simulink model "IdentPlanar"  (Simulink 7.9)
settings: Solver=FixedStepDiscrete  StartTime=0.0  StopTime=3600  FixedStep=1/Fs  RelTol=1e-3
values from neighbouring files (symbols this model uses):
  abs2deg_s1 = (s1max-s1min)/(s1maxabs-s1minabs)    (= 0.280034572169)    [Alex_init_const_wrist.m]
  abs2deg_s2 = (s2max-s2min)/(s2maxabs-s2minabs)    (= 0.060826446281)    [Alex_init_const_wrist.m]
  c1x = 0    [Alex_init_const_shoulderelbow.m]
  c1y = 0    [Alex_init_const_shoulderelbow.m]
  c1z = 0    [Alex_init_const_shoulderelbow.m]
  c2x = 1.79e-3    (= 0.00179)    [Alex_init_const_shoulderelbow.m]
  c2y = 0    [Alex_init_const_shoulderelbow.m]
  c2z = 228.5e-3    (= 0.2285)    [Alex_init_const_shoulderelbow.m]
  c3x = 0    [Alex_init_const_shoulderelbow.m]
  c3y = 0    [Alex_init_const_shoulderelbow.m]
  c3z = 0    [Alex_init_const_shoulderelbow.m]
  c4x = 1.91e-3    (= 0.00191)    [Alex_init_const_shoulderelbow.m]
  c4y = 0    [Alex_init_const_shoulderelbow.m]
  c4z = 163e-3    (= 0.163)    [Alex_init_const_shoulderelbow.m]
  c5x = 0    [Alex_init_const_shoulderelbow.m]
  c5y = 0    [Alex_init_const_shoulderelbow.m]
  c5z = 0    [Alex_init_const_shoulderelbow.m]
  deg_rad = pi/180    (= 0.0174532925199)    [Alex_init_const_shoulderelbow.m]
  E1initial = qtot(initialtime*Fs,1)    [Alex_init_const_shoulderelbow.m]
  Fs = 1000    [Alex_init_const_wrist.m]
  initialtime = 5    [Alex_init_const_shoulderelbow.m]
  Ll = 324.6e-3    (= 0.3246)    [Alex_init_const_shoulderelbow.m]
  Lu = 332.3e-3    (= 0.3323)    [Alex_init_const_shoulderelbow.m]
  ml = 1.649    [Alex_init_const_shoulderelbow.m]
  mu = 2.804    [Alex_init_const_shoulderelbow.m]
  Nm2mA_e1 = 1000/(Kv_e1*GRe1)    [Alex_init_const_shoulderelbow.m]
  Nm2mA_s1 = 1000/(Kv_s1*GR_s1)    [Alex_init_const_shoulderelbow.m]
  Nm2mA_s2 = 1000/(Kv_s2*GR_s2)    [Alex_init_const_shoulderelbow.m]
  Nm2mA_s3 = 1000/(Kv_s3*GR_s3)    [Alex_init_const_shoulderelbow.m]
  S2initial = qtot(initialtime*Fs,2)    [Alex_init_const_shoulderelbow.m]
  s2maxabs = 3420    [Alex_init_const_wrist.m]
  s2minabs = 395    [Alex_init_const_wrist.m]
  Ts = 1/Fs    [Alex_init_const_shoulderelbow.m]    (also in Alex_init_const_wrist.m = 0.001)
undefined symbols (not defined in the file or in its folder): abs2deg_e1, abs2deg_e2, abs2deg_s3, CPT_s1, CPT_s2, CPTe1, CPTe2, CPTs3, e2maxabs, e2minabs, GR_s1, GR_s2, GR_s3, GRe1, GRe2, ilim_e1, ilim_e2, ilim_s1, ilim_s2, ilim_s3, Kd_e1, Kd_e2, Kd_s1, Kd_s2, Kd_s3, Ki_e1, Ki_e2, Ki_s1, Ki_s2, Ki_s3, s1zeroabs, s3maxabs, s3minabs
libraries: SERGIOarm x10, simulink x4, SERGIO_Lib x2
settings Model: Creator=root  LastModifiedBy=root  SimulationMode=external  ExtModeTrigElement=1  ExtModeTrigDuration=3910  ExtModeAutoUpdateStatusClock=off
settings DataIOCC: LimitDataPoints=off  MaxDataPoints=4000*3600  SaveOutput=off  SignalLogging=off  SaveTime=off
settings OptimizationCC: BlockReduction=off  BooleanDataType=off  InitFltsAndDblsToZero=on
settings DebuggingCC: SaveWithParameterizedLinksMsg=none  SignalResolutionControl=TryResolveAllWithWarning  SolverPrmCheckMsg=none  MultiTaskDSMMsg=warning  MultiTaskCondExecSysMsg=none  FcnCallInpInsideContextMsg=Use local settings  StrictBusMsg=None
settings HardwareCC: TargetBitPerLong=64  TargetBitPerPointer=64  TargetEndianess=LittleEndian  TargetWordSize=64  TargetHWDeviceType=MATLAB Host
settings ModelReferenceCC: ModelReferencePassRootInputsByReference=off
settings RTWCC: SystemTargetFile=mttarget.tlc  MakeCommand="make_rtw CC=\"ccache gcc\" OPTS=\"-DNETIF_ID=0 -D_GNU_SOURCE -DPRIO=99\""  TemplateMakefile=mt_unix.tmf  Description=Robocup Real-Time Motion Target  ProcessScript=mttarget_make_rtw_hook  IncludeERTFirstTime=on  RTWCompilerOptimization=Custom  RTWCustomCompilerOptimizations=-O2 -g -W
settings RTWCC: CustomInclude=|
  | /usr/local/include/soem
  | /usr/local/include/timer_posix
settings RTWCC: CustomLibrary=|
  | /usr/local/lib/libsoem.so
  | /usr/lib/libtimer_posix.so
settings GRTTargetCC: LogVarNameModifier=none  ExtMode=on

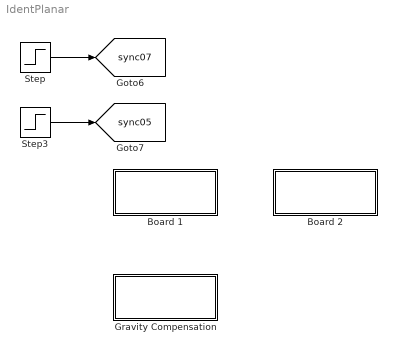
== system IdentPlanar ==
  Board 1 : Subsystem
  Board 2 : Subsystem
  Gravity Compensation : Subsystem
  Step : Step  Time=0.7  Before=1  After=0  SampleTime=0
  Step3 : Step  Time=0.5  Before=1  After=0  SampleTime=0
  tag scope: sync05=global, sync07=global
  wires:
  Step/1 -> [sync07]
  Step3/1 -> [sync05]

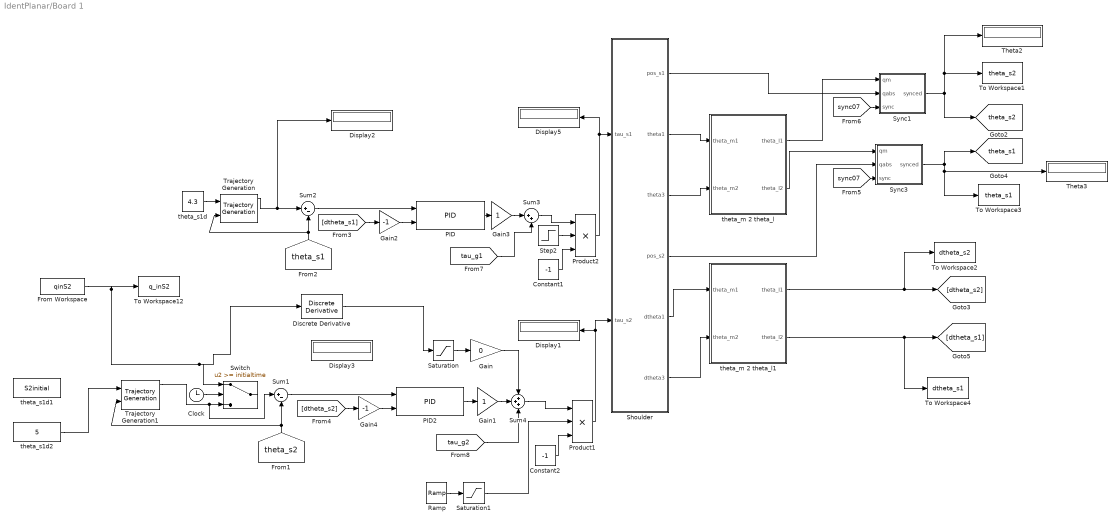
== system IdentPlanar/Board 1 ==
  Clock : Clock
  Constant1 : Constant  Value=-1
  Constant2 : Constant  Value=-1
  Discrete Derivative : simulink/Discrete/Discrete Derivative  gainval=1.0  ICPrevScaledInput=0.0  InputProcessing=Inherited  OutMin=[]  OutMax=[]  OutDataType=fixdt(1, 16)  OutScaling=2^-10  DoSatur=off
  Display{1..3,5} (4 alike) : Display
  From Workspace : FromWorkspace  VariableName=qinS2  SampleTime=1/Fs  OutputAfterFinalValue=Holding final value
  Gain : Gain  Gain=0
  Gain1 : Gain
  Gain2 : Gain  Gain=-1
  Gain3 : Gain
  Gain4 : Gain  Gain=-1
  PID : SERGIOarm/PID  Kc=Kc_s1  Ki=Ki_s1  Kd=Kd_s1  uplim=ilim_s1  lowlim=-ilim_s1  Ts=Ts
  PID2 : SERGIOarm/PID  Kc=Kc_s2  Ki=Ki_s2  Kd=Kd_s2  uplim=ilim_s2  lowlim=-ilim_s2  Ts=Ts
  Product1 : Product  Inputs=3  RndMeth=Zero
  Product2 : Product  Inputs=3  RndMeth=Zero
  Ramp : simulink/Sources/Ramp  slope=1  start=0.8  X0=0
  Saturation : Saturate  UpperLimit=1  LowerLimit=-1
  Saturation1 : Saturate  UpperLimit=1  LowerLimit=0
  Shoulder : Subsystem
  Step2 : Step  Time=0.8  SampleTime=0
  Sum1 : Sum  Inputs=|+-
  Sum2 : Sum  Inputs=|+-
  Sum3 : Sum  Inputs=|++
  Sum4 : Sum  Inputs=+++
  Switch : Switch  Threshold=initialtime
  Sync1 : Subsystem
  Sync3 : Subsystem
  Theta2 : Display
  Theta3 : Display
  To Workspace1 : ToWorkspace  VariableName=theta_s2  SampleTime=-1
  To Workspace12 : ToWorkspace  VariableName=q_inS2  SampleTime=-1
  To Workspace2 : ToWorkspace  VariableName=dtheta_s2  SampleTime=-1
  To Workspace3 : ToWorkspace  VariableName=theta_s1  SampleTime=-1
  To Workspace4 : ToWorkspace  VariableName=dtheta_s1  SampleTime=-1
  Trajectory Generation : SERGIOarm/Trajectory Generation  Vmax=Vmax  Amax=Amax  dif_in=0.1
  Trajectory Generation1 : SERGIOarm/Trajectory Generation  Vmax=Vmax  Amax=Amax  dif_in=1
  theta_m 2 theta_l : Subsystem
  theta_m 2 theta_l1 : Subsystem
  theta_s1d : Constant  Value=4.3
  theta_s1d1 : Constant  Value=S2initial
  theta_s1d2 : Constant  Value=5
  tag scope: theta_s1=global, theta_s2=global
  wires:
  Product2/1 -> Display5/1, Shoulder/1(tau_s1)
  theta_m 2 theta_l/1(theta_l1) -> Sync1/1(qm)
  theta_m 2 theta_l/2(theta_l2) -> Sync3/1(qm)
  Shoulder/6(dtheta3) -> theta_m 2 theta_l1/2(theta_m2)
  theta_m 2 theta_l1/1(theta_l1) -> [dtheta_s2], To Workspace2/1
  theta_m 2 theta_l1/2(theta_l2) -> [dtheta_s1], To Workspace4/1
  Step2/1 -> Product2/2
  Constant1/1 -> Product2/3
  [dtheta_s1] -> Gain2/1
  Product1/1 -> Display1/1, Shoulder/2(tau_s2)
  Saturation1/1 -> Product1/2
  Constant2/1 -> Product1/3
  [dtheta_s2] -> Gain4/1
  Shoulder/5(dtheta1) -> theta_m 2 theta_l1/1(theta_m1)
  Shoulder/2(theta1) -> theta_m 2 theta_l/1(theta_m1)
  Shoulder/3(theta3) -> theta_m 2 theta_l/2(theta_m2)
  Shoulder/4(pos_s2) -> Sync3/2(qabs)
  Sync3/1(synced) -> [theta_s1], Theta3/1, To Workspace3/1
  [sync07] -> Sync3/3(sync)
  Shoulder/1(pos_s1) -> Sync1/2(qabs)
  [sync07] -> Sync1/3(sync)
  Sync1/1(synced) -> [theta_s2], To Workspace1/1, Theta2/1
  Gain3/1 -> Sum3/1
  [tau_g1] -> Sum3/2
  PID/1 -> Gain3/1
  Sum3/1 -> Product2/1
  PID2/1 -> Gain1/1
  Sum4/1 -> Product1/1
  Trajectory Generation/1 -> Sum2/1, Display2/1
  Sum2/1 -> PID/1
  [theta_s1] -> Sum2/2, Trajectory Generation/2
  theta_s1d/1 -> Trajectory Generation/1
  Sum1/1 -> PID2/1
  [theta_s2] -> Sum1/2, Trajectory Generation1/2
  Gain2/1 -> PID/2
  Gain4/1 -> PID2/2
  From Workspace/1 -> To Workspace12/1, Discrete Derivative/1, Switch/1
  Discrete Derivative/1 -> Saturation/1
  Saturation/1 -> Gain/1
  Gain/1 -> Sum4/1
  Gain1/1 -> Sum4/2
  [tau_g2] -> Sum4/3
  Trajectory Generation1/1 -> Switch/3, Sum1/1
  Clock/1 -> Switch/2
  Ramp/1 -> Saturation1/1
  theta_s1d2/1 -> Trajectory Generation1/1

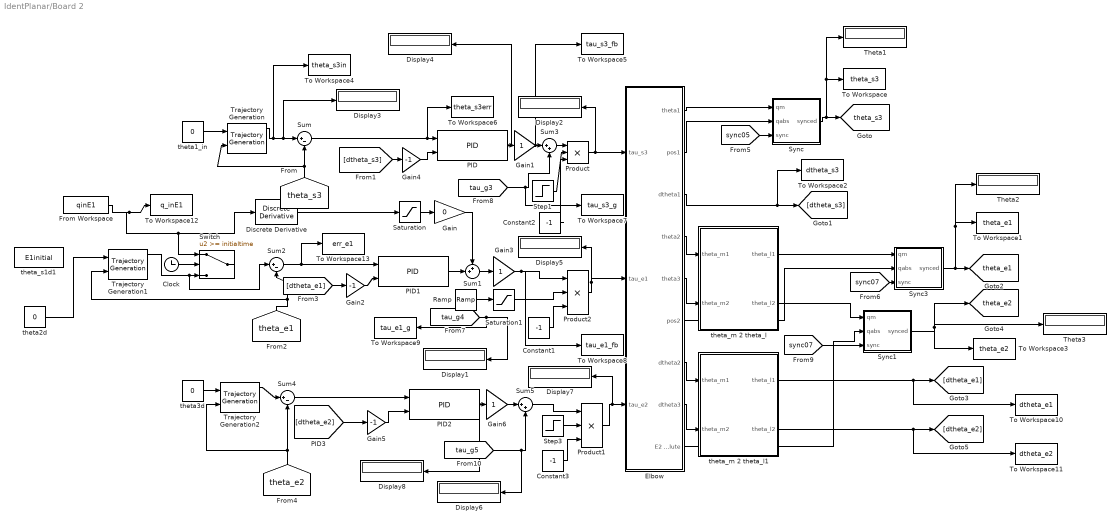
== system IdentPlanar/Board 2 ==
  Clock : Clock
  Constant1 : Constant  Value=-1
  Constant2 : Constant  Value=-1
  Constant3 : Constant  Value=-1
  Discrete Derivative : simulink/Discrete/Discrete Derivative  gainval=1.0  ICPrevScaledInput=0.0  InputProcessing=Inherited  OutMin=[]  OutMax=[]  OutDataType=fixdt(1, 16)  OutScaling=2^-10  DoSatur=off
  Display{1..8} (8 alike) : Display
  Elbow : Subsystem
  From Workspace : FromWorkspace  VariableName=qinE1  SampleTime=1/Fs  OutputAfterFinalValue=Holding final value
  Gain : Gain  Gain=0
  Gain1 : Gain
  Gain2 : Gain  Gain=-1
  Gain3 : Gain
  Gain4 : Gain  Gain=-1
  Gain5 : Gain  Gain=-1
  Gain6 : Gain
  PID : SERGIOarm/PID  Kc=Kc_s3  Ki=Ki_s3  Kd=Kd_s3  uplim=ilim_s3  lowlim=-ilim_s3  Ts=Ts
  PID1 : SERGIOarm/PID  Kc=Kc_e1  Ki=Ki_e1  Kd=Kd_e1  uplim=ilim_e1  lowlim=-ilim_e1  Ts=Ts
  PID2 : SERGIOarm/PID  Kc=Kc_e2  Ki=Ki_e2  Kd=Kd_e2  uplim=ilim_e2  lowlim=-ilim_e2  Ts=Ts
  Product : Product  Inputs=3  RndMeth=Zero
  Product1 : Product  Inputs=3  RndMeth=Zero
  Product2 : Product  Inputs=3  RndMeth=Zero
  Ramp : simulink/Sources/Ramp  slope=1  start=0.8  X0=0
  Saturation : Saturate  UpperLimit=1  LowerLimit=-1
  Saturation1 : Saturate  UpperLimit=1  LowerLimit=0
  Step1 : Step  Time=0.8  SampleTime=0
  Step3 : Step  Time=0.8  SampleTime=0
  Sum : Sum  Inputs=|+-
  Sum1 : Sum  Inputs=++|
  Sum2 : Sum  Inputs=|+-
  Sum3 : Sum  Inputs=|++
  Sum4 : Sum  Inputs=|+-
  Sum5 : Sum  Inputs=|++
  Switch : Switch  Threshold=initialtime
  Sync : Subsystem
  Sync1 : Subsystem
  Sync3 : Subsystem
  Theta1 : Display
  Theta2 : Display
  Theta3 : Display
  To Workspace : ToWorkspace  VariableName=theta_s3  SampleTime=-1
  To Workspace1 : ToWorkspace  VariableName=theta_e1  SampleTime=-1
  To Workspace10 : ToWorkspace  VariableName=dtheta_e1  SampleTime=-1
  To Workspace11 : ToWorkspace  VariableName=dtheta_e2  SampleTime=-1
  To Workspace12 : ToWorkspace  VariableName=q_inE1  SampleTime=-1
  To Workspace13 : ToWorkspace  VariableName=err_e1  SampleTime=-1
  To Workspace2 : ToWorkspace  VariableName=dtheta_s3  SampleTime=-1
  To Workspace3 : ToWorkspace  VariableName=theta_e2  SampleTime=-1
  To Workspace4 : ToWorkspace  VariableName=theta_s3in  SampleTime=-1
  To Workspace5 : ToWorkspace  VariableName=tau_s3_fb  SampleTime=-1
  To Workspace6 : ToWorkspace  VariableName=theta_s3err  SampleTime=-1
  To Workspace7 : ToWorkspace  VariableName=tau_s3_g  SampleTime=-1
  To Workspace8 : ToWorkspace  VariableName=tau_e1_fb  SampleTime=-1
  To Workspace9 : ToWorkspace  VariableName=tau_e1_g  SampleTime=-1
  Trajectory Generation : SERGIOarm/Trajectory Generation  Vmax=Vmax  Amax=Amax  dif_in=1
  Trajectory Generation1 : SERGIOarm/Trajectory Generation  Vmax=Vmax  Amax=Amax  dif_in=0.1
  Trajectory Generation2 : SERGIOarm/Trajectory Generation  Vmax=Vmax  Amax=Amax  dif_in=1
  theta1_in : Constant  Value=0
  theta2d : Constant  Value=0
  theta3d : Constant  Value=0
  theta_m 2 theta_l : Subsystem
  theta_m 2 theta_l1 : Subsystem
  theta_s1d1 : Constant  Value=E1initial
  tag scope: theta_e1=global, theta_e2=global, theta_s3=global
  wires:
  [theta_s3] -> Sum/2, Trajectory Generation/2
  [theta_e1] -> Sum2/2, Trajectory Generation1/2
  Sum4/1 -> PID2/1
  [theta_e2] -> Sum4/2, Trajectory Generation2/2
  Elbow/1(theta1) -> Sync/1(qm)
  Step1/1 -> Product/2
  [sync05] -> Sync/3(sync)
  Sum/1 -> To Workspace6/1, PID/1
  Product2/1 -> Elbow/2(tau_e1), Display5/1
  [dtheta_s3] -> Gain4/1
  Product/1 -> Elbow/1(tau_s3), Display2/1
  Sync/1(synced) -> [theta_s3], To Workspace/1, Theta1/1
  Elbow/2(pos1) -> Sync/2(qabs)
  Elbow/3(dtheta1) -> [dtheta_s3], To Workspace2/1
  Elbow/4(theta2) -> theta_m 2 theta_l/1(theta_m1)
  Elbow/5(theta3) -> theta_m 2 theta_l/2(theta_m2)
  theta_m 2 theta_l/1(theta_l1) -> Sync3/1(qm)
  Elbow/6(pos2) -> Sync3/2(qabs)
  Sync3/1(synced) -> [theta_e1], To Workspace1/1, Theta2/1
  [sync07] -> Sync3/3(sync)
  Elbow/7(dtheta2) -> theta_m 2 theta_l1/1(theta_m1)
  Elbow/8(dtheta3) -> theta_m 2 theta_l1/2(theta_m2)
  theta_m 2 theta_l1/1(theta_l1) -> [dtheta_e1], To Workspace10/1
  theta_m 2 theta_l1/2(theta_l2) -> [dtheta_e2], To Workspace11/1
  Saturation1/1 -> Product2/2
  Constant1/1 -> Product2/3
  [dtheta_e1] -> Gain2/1
  Gain3/1 -> To Workspace8/1, Product2/1
  PID/1 -> Gain1/1, Display4/1
  Gain1/1 -> Sum3/1, To Workspace5/1
  Sum3/1 -> Product/1
  [tau_g3] -> Sum3/2, To Workspace7/1
  Sum2/1 -> PID1/1, To Workspace13/1
  Constant2/1 -> Product/3
  theta1_in/1 -> Trajectory Generation/1
  Gain2/1 -> PID1/2
  Gain4/1 -> PID/2
  theta_m 2 theta_l/2(theta_l2) -> Sync1/1(qm)
  Elbow/9(E2 absolute) -> Sync1/2(qabs)
  [sync07] -> Sync1/3(sync)
  Sync1/1(synced) -> [theta_e2], To Workspace3/1, Theta3/1
  Trajectory Generation2/1 -> Sum4/1
  theta3d/1 -> Trajectory Generation2/1
  Gain5/1 -> PID2/2
  [dtheta_e2] -> Gain5/1
  Step3/1 -> Product1/2
  Constant3/1 -> Product1/3
  Sum5/1 -> Product1/1
  Gain6/1 -> Sum5/1
  [tau_g5] -> Sum5/2, Display6/1
  PID2/1 -> Gain6/1, Display8/1
  Product1/1 -> Elbow/3(tau_e2), Display7/1
  Trajectory Generation/1 -> To Workspace4/1, Sum/1, Display3/1
  From Workspace/1 -> To Workspace12/1, Discrete Derivative/1, Switch/1
  [tau_g4] -> To Workspace9/1, Display1/1
  Saturation/1 -> Gain/1
  Sum1/1 -> Gain3/1
  PID1/1 -> Sum1/2
  Discrete Derivative/1 -> Saturation/1
  Gain/1 -> Sum1/1
  Trajectory Generation1/1 -> Switch/3, Sum2/1
  Clock/1 -> Switch/2
  Ramp/1 -> Saturation1/1
  theta2d/1 -> Trajectory Generation1/1

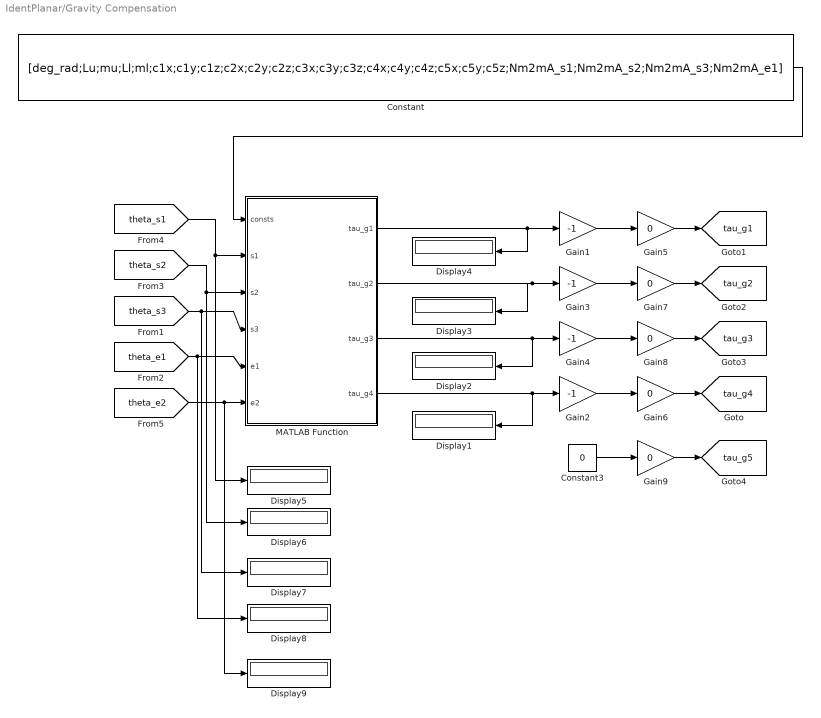
== system IdentPlanar/Gravity Compensation ==
  Constant : Constant  Value=[deg_rad;Lu;mu;Ll;ml;c1x;c1y;c1z;c2x;c2y;c2z;c3x;c3y;c3z;c4x;c4y;c4z;c5x;c5y;c5z;Nm2mA_s1;Nm2mA_s2;Nm2mA_s3;Nm2mA_e1]
  Constant3 : Constant  Value=0
  Display{1..9} (9 alike) : Display
  Gain{1..4} (4 alike) : Gain  Gain=-1
  Gain{5..9} (5 alike) : Gain  Gain=0
  MATLAB Function : MATLAB Function  TreatAsAtomicUnit=on
  tag scope: tau_g1=global, tau_g2=global, tau_g3=global, tau_g4=global, tau_g5=global
  wires:
  [theta_s1] -> Display5/1, MATLAB Function/2(s1)
  [theta_s2] -> Display6/1, MATLAB Function/3(s2)
  [theta_s3] -> MATLAB Function/4(s3), Display7/1
  [theta_e1] -> MATLAB Function/5(e1), Display8/1
  [theta_e2] -> MATLAB Function/6(e2), Display9/1
  Constant/1 -> MATLAB Function/1(consts)
  MATLAB Function/1(tau_g1) -> Display4/1, Gain1/1
  MATLAB Function/2(tau_g2) -> Display3/1, Gain3/1
  MATLAB Function/3(tau_g3) -> Display2/1, Gain4/1
  MATLAB Function/4(tau_g4) -> Display1/1, Gain2/1
  Gain1/1 -> Gain5/1
  Gain3/1 -> Gain7/1
  Gain4/1 -> Gain8/1
  Gain2/1 -> Gain6/1
  Gain5/1 -> [tau_g1]
  Gain7/1 -> [tau_g2]
  Gain8/1 -> [tau_g3]
  Gain6/1 -> [tau_g4]
  Gain9/1 -> [tau_g5]
  Constant3/1 -> Gain9/1

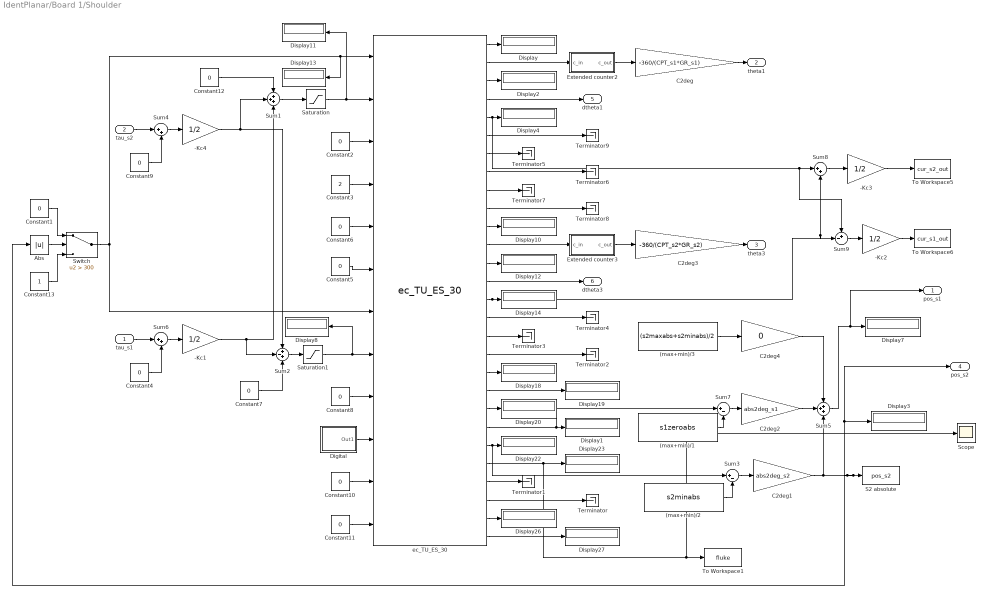
== system IdentPlanar/Board 1/Shoulder ==
  tau_s1 : Inport
  tau_s2 : Inport  Port=2
  (max+min)/1 : Constant  Value=s1zeroabs
  (max+min)/2 : Constant  Value=s2minabs
  (max+min)/3 : Constant  Value=(s2maxabs+s2minabs)/2
  -Kc{1..4} (4 alike) : Gain  Gain=1/2
  Abs : Abs
  C2deg : Gain  Gain=-360/(CPT_s1*GR_s1)
  C2deg1 : Gain  Gain=abs2deg_s2
  C2deg2 : Gain  Gain=abs2deg_s1
  C2deg3 : Gain  Gain=-360/(CPT_s2*GR_s2)
  C2deg4 : Gain  Gain=0
  Constant{1..2,4..12} (11 alike) : Constant  Value=0
  Constant13 : Constant
  Constant3 : Constant  Value=2
  Digital : Subsystem
  Display{,1..4,7..8,10..14,18..20,22..23,26..27} (19 alike) : Display
  Extended counter2 : Subsystem
  Extended counter3 : Subsystem
  S2 absolute : ToWorkspace  VariableName=pos_s2  SampleTime=-1
  Saturation : Saturate  UpperLimit=2400  LowerLimit=-2400
  Saturation1 : Saturate  UpperLimit=2400  LowerLimit=-2400
  Scope : Scope
      settings: TimeRange=10  YMin=0  YMax=350  SampleInput=on
  Sum1 : Sum  Inputs=+++
  Sum2 : Sum  Inputs=+-+
  Sum3 : Sum  Inputs=|+-
  Sum4 : Sum  Inputs=|++
  Sum5 : Sum  Inputs=+++
  Sum6 : Sum  Inputs=|++
  Sum7 : Sum  Inputs=|+-
  Sum8 : Sum  Inputs=|++
  Sum9 : Sum  Inputs=+-|
  Switch : Switch  Criteria=u2 > Threshold  Threshold=300
  Terminator{,1..9} (10 alike) : Terminator
  To Workspace1 : ToWorkspace  VariableName=fluke  SampleTime=-1
  To Workspace5 : ToWorkspace  VariableName=cur_s2_out  SampleTime=-1
  To Workspace6 : ToWorkspace  VariableName=cur_s1_out  SampleTime=-1
  ec_TU_ES_30 : SERGIO_Lib/EtherCAT Blocks/ec_TU_ES_30  link_id=1  slave_num=2  resistance=[0.611+0.45*2, 1.0, 0.611+0.45*2]  kv=[0.0259, 0, 0.0259]  pgain=[4.00, 0.00, 4.00]  igain=[50.00, 0.00, 50.00]  ilimit=[1.0, 1.0, 1.0]  encdir=[1, 1, 1]  encres=[2000, 2000, 2000]  czero=[17230, 8633, 8526]
  pos_s1 : Outport
  theta1 : Outport  Port=2
  theta3 : Outport  Port=3
  pos_s2 : Outport  Port=4
  dtheta1 : Outport  Port=5
  dtheta3 : Outport  Port=6
  wires:
  Constant2/1 -> ec_TU_ES_30/3
  Constant5/1 -> ec_TU_ES_30/6
  Constant8/1 -> ec_TU_ES_30/9
  Digital/1(Out1) -> ec_TU_ES_30/10
  Constant10/1 -> ec_TU_ES_30/11
  Constant11/1 -> ec_TU_ES_30/12
  ec_TU_ES_30/1 -> Display/1
  ec_TU_ES_30/3 -> Display2/1
  ec_TU_ES_30/4 -> dtheta1/1
  ec_TU_ES_30/5 -> Display4/1, Sum8/1, Sum9/1
  ec_TU_ES_30/6 -> Terminator9/1
  ec_TU_ES_30/8 -> Terminator6/1
  ec_TU_ES_30/9 -> Terminator7/1
  ec_TU_ES_30/10 -> Terminator8/1
  ec_TU_ES_30/11 -> Display10/1
  ec_TU_ES_30/13 -> Display12/1
  ec_TU_ES_30/14 -> dtheta3/1
  ec_TU_ES_30/15 -> Display14/1, Sum8/2, Sum9/2
  ec_TU_ES_30/16 -> Terminator4/1
  ec_TU_ES_30/17 -> Terminator3/1
  ec_TU_ES_30/18 -> Terminator2/1
  ec_TU_ES_30/19 -> Display18/1
  ec_TU_ES_30/20 -> Display19/1
  ec_TU_ES_30/21 -> Display20/1
  ec_TU_ES_30/24 -> Display23/1, To Workspace1/1, Scope/1
  ec_TU_ES_30/25 -> Terminator1/1
  ec_TU_ES_30/26 -> Terminator/1
  ec_TU_ES_30/27 -> Display26/1
  ec_TU_ES_30/28 -> Display27/1
  C2deg/1 -> theta1/1
  ec_TU_ES_30/2 -> Extended counter2/1(c_in)
  Extended counter2/1(c_out) -> C2deg/1
  Sum1/1 -> Saturation/1
  Saturation/1 -> ec_TU_ES_30/2, Display11/1
  Sum2/1 -> Saturation1/1
  Saturation1/1 -> ec_TU_ES_30/8, Display8/1
  ec_TU_ES_30/7 -> Terminator5/1
  ec_TU_ES_30/12 -> Extended counter3/1(c_in)
  Extended counter3/1(c_out) -> C2deg3/1
  C2deg3/1 -> theta3/1
  Sum4/1 -> -Kc4/1
  tau_s2/1 -> Sum4/1
  Sum6/1 -> -Kc1/1
  tau_s1/1 -> Sum6/1
  Constant4/1 -> Sum6/2
  ec_TU_ES_30/22 -> Display1/1, Sum7/1
  Constant3/1 -> ec_TU_ES_30/4
  Constant6/1 -> ec_TU_ES_30/5
  Constant12/1 -> Sum1/1
  -Kc4/1 -> Sum1/2, Sum2/1
  -Kc1/1 -> Sum1/3, Sum2/2
  Constant9/1 -> Sum4/2
  Constant7/1 -> Sum2/3
  (max+min)/2/1 -> Sum3/2
  Sum3/1 -> C2deg1/1
  C2deg1/1 -> S2 absolute/1, Abs/1, Display3/1, pos_s2/1, Sum5/3
  ec_TU_ES_30/23 -> Display22/1, Sum3/1
  Switch/1 -> ec_TU_ES_30/7, ec_TU_ES_30/1, Display13/1
  Constant1/1 -> Switch/1
  Abs/1 -> Switch/2
  Constant13/1 -> Switch/3
  Sum5/1 -> Display7/1, pos_s1/1
  (max+min)/3/1 -> C2deg4/1
  C2deg4/1 -> Sum5/1
  C2deg2/1 -> Sum5/2
  (max+min)/1/1 -> Sum7/2
  Sum7/1 -> C2deg2/1
  Sum8/1 -> -Kc3/1
  -Kc3/1 -> To Workspace5/1
  Sum9/1 -> -Kc2/1
  -Kc2/1 -> To Workspace6/1

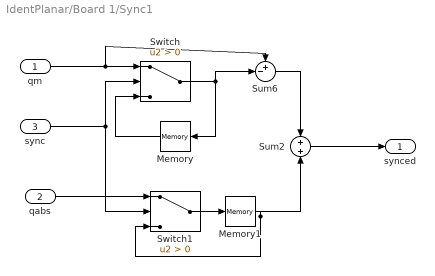
== system IdentPlanar/Board 1/Sync1 ==
  qm : Inport
  qabs : Inport  Port=2
  sync : Inport  Port=3
  Memory : Memory
  Memory1 : Memory
  Sum2 : Sum
  Sum6 : Sum  Inputs=+-|
  Switch : Switch  Criteria=u2 > Threshold
  Switch1 : Switch  Criteria=u2 > Threshold
  synced : Outport
  wires:
  Switch/1 -> Sum6/2, Memory/1
  Memory/1 -> Switch/3
  qm/1 -> Switch/1, Sum6/1
  Sum6/1 -> Sum2/1
  Sum2/1 -> synced/1
  sync/1 -> Switch/2, Switch1/2
  Memory1/1 -> Switch1/3, Sum2/2
  Switch1/1 -> Memory1/1
  qabs/1 -> Switch1/1

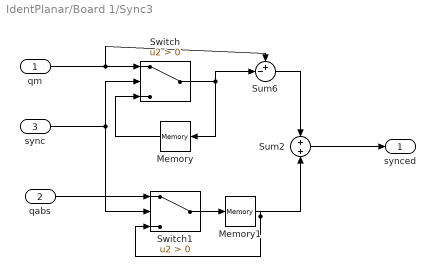
== system IdentPlanar/Board 1/Sync3 ==
  qm : Inport
  qabs : Inport  Port=2
  sync : Inport  Port=3
  Memory : Memory
  Memory1 : Memory
  Sum2 : Sum
  Sum6 : Sum  Inputs=+-|
  Switch : Switch  Criteria=u2 > Threshold
  Switch1 : Switch  Criteria=u2 > Threshold
  synced : Outport
  wires:
  Switch/1 -> Sum6/2, Memory/1
  Memory/1 -> Switch/3
  qm/1 -> Switch/1, Sum6/1
  Sum6/1 -> Sum2/1
  Sum2/1 -> synced/1
  sync/1 -> Switch/2, Switch1/2
  Memory1/1 -> Switch1/3, Sum2/2
  Switch1/1 -> Memory1/1
  qabs/1 -> Switch1/1

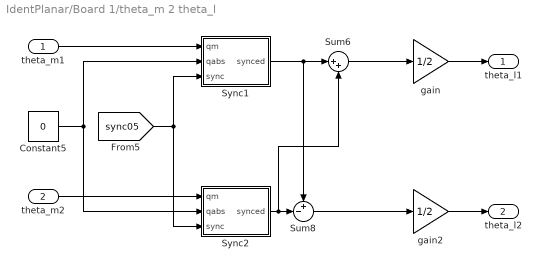
== system IdentPlanar/Board 1/theta_m 2 theta_l ==
  theta_m1 : Inport
  theta_m2 : Inport  Port=2
  Constant5 : Constant  Value=0
  Sum6 : Sum  Inputs=|++
  Sum8 : Sum  Inputs=+-|
  Sync1 : Subsystem
  Sync2 : Subsystem
  gain : Gain  Gain=1/2
  gain2 : Gain  Gain=1/2
  theta_l1 : Outport
  theta_l2 : Outport  Port=2
  wires:
  theta_m2/1 -> Sync2/1(qm)
  theta_m1/1 -> Sync1/1(qm)
  Constant5/1 -> Sync1/2(qabs), Sync2/2(qabs)
  Sync2/1(synced) -> Sum8/2, Sum6/2
  Sync1/1(synced) -> Sum6/1, Sum8/1
  Sum6/1 -> gain/1
  gain/1 -> theta_l1/1
  gain2/1 -> theta_l2/1
  [sync05] -> Sync1/3(sync), Sync2/3(sync)
  Sum8/1 -> gain2/1

== system IdentPlanar/Board 1/theta_m 2 theta_l1 ==
  theta_m1 : Inport
  theta_m2 : Inport  Port=2
  Sum6 : Sum  Inputs=|++
  Sum8 : Sum  Inputs=+-|
  gain : Gain  Gain=-1/2
  gain2 : Gain  Gain=-1/2
  theta_l1 : Outport
  theta_l2 : Outport  Port=2
  wires:
  Sum6/1 -> gain/1
  gain/1 -> theta_l1/1
  Sum8/1 -> gain2/1
  gain2/1 -> theta_l2/1
  theta_m1/1 -> Sum6/1, Sum8/1
  theta_m2/1 -> Sum6/2, Sum8/2

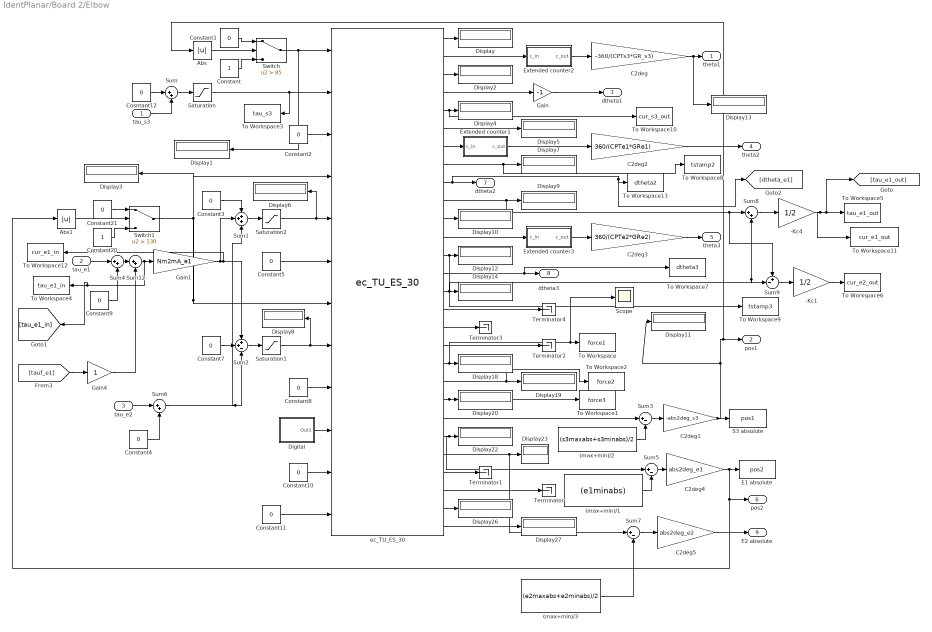
== system IdentPlanar/Board 2/Elbow ==
  tau_s3 : Inport
  tau_e1 : Inport  Port=2
  tau_e2 : Inport  Port=3
  (max+min)/1 : Constant  Value=(e1minabs)
  (max+min)/2 : Constant  Value=(s3maxabs+s3minabs)/2
  (max+min)/3 : Constant  Value=(e2maxabs+e2minabs)/2
  -Kc1 : Gain  Gain=1/2
  -Kc4 : Gain  Gain=1/2
  Abs : Abs
  Abs1 : Abs
  C2deg : Gain  Gain=-360/(CPTs3*GR_s3)
  C2deg1 : Gain  Gain=-abs2deg_s3
  C2deg2 : Gain  Gain=360/(CPTe1*GRe1)
  C2deg3 : Gain  Gain=360/(CPTe2*GRe2)
  C2deg4 : Gain  Gain=abs2deg_e1
  C2deg5 : Gain  Gain=abs2deg_e2
  Constant : Constant
  Constant{1..5,7..11,21} (11 alike) : Constant  Value=0
  Constant20 : Constant
  Cosntant12 : Constant  Value=0
  Digital : Subsystem
  Display{,1..14,18..20,22..23,26..27} (22 alike) : Display
  E1 absolute : ToWorkspace  VariableName=pos2  SampleTime=-1
  Extended counter1 : Subsystem
  Extended counter2 : Subsystem
  Extended counter3 : Subsystem
  Gain : Gain  Gain=-1
  Gain1 : Gain  Gain=Nm2mA_e1
  Gain4 : Gain
  S3 absolute : ToWorkspace  VariableName=pos1  SampleTime=-1
  Saturation : Saturate  UpperLimit=3400  LowerLimit=-3400
  Saturation1 : Saturate  UpperLimit=1400  LowerLimit=-1400
  Saturation2 : Saturate  UpperLimit=1400  LowerLimit=-1400
  Scope : Scope
      settings: TimeRange=5  YMin=1050  YMax=1150  SaveName=force1scope
  Sum{,4,6,8,12} (5 alike) : Sum  Inputs=|++
  Sum1 : Sum  Inputs=+++
  Sum2 : Sum  Inputs=++-
  Sum3 : Sum  Inputs=|+-
  Sum5 : Sum  Inputs=|+-
  Sum7 : Sum  Inputs=|+-
  Sum9 : Sum  Inputs=+-|
  Switch : Switch  Criteria=u2 > Threshold  Threshold=85
  Switch1 : Switch  Criteria=u2 > Threshold  Threshold=130
  Terminator{,1..4} (5 alike) : Terminator
  To Workspace : ToWorkspace  VariableName=force1  SampleTime=-1
  To Workspace1 : ToWorkspace  VariableName=force3  SampleTime=-1
  To Workspace10 : ToWorkspace  VariableName=cur_s3_out  SampleTime=-1
  To Workspace11 : ToWorkspace  VariableName=cur_e1_out  SampleTime=-1
  To Workspace12 : ToWorkspace  VariableName=cur_e1_in  SampleTime=-1
  To Workspace13 : ToWorkspace  VariableName=dtheta2  SampleTime=-1
  To Workspace2 : ToWorkspace  VariableName=force2  SampleTime=-1
  To Workspace3 : ToWorkspace  VariableName=tau_s3  SampleTime=-1
  To Workspace4 : ToWorkspace  VariableName=tau_e1_in  SampleTime=-1
  To Workspace5 : ToWorkspace  VariableName=tau_e1_out  SampleTime=-1
  To Workspace6 : ToWorkspace  VariableName=cur_e2_out  SampleTime=-1
  To Workspace7 : ToWorkspace  VariableName=dtheta3  SampleTime=-1
  To Workspace8 : ToWorkspace  VariableName=tstamp2  SampleTime=-1
  To Workspace9 : ToWorkspace  VariableName=tstamp3  SampleTime=-1
  ec_TU_ES_30 : SERGIO_Lib/EtherCAT Blocks/ec_TU_ES_30  link_id=2  slave_num=3  resistance=[1.511, 1.53+0.45*2, 1.53+0.45*2]  kv=[0.0259, 0.0208, 0.0208]  pgain=[4.00, 4.00, 4.00]  igain=[50.00, 50.00, 50.00]  ilimit=[1.0, 1.0, 1.0]  encdir=[1, 1, 1]  encres=[2000, 500, 500]  czero=[17330, 8633, 8522]
  theta1 : Outport
  pos1 : Outport  Port=2
  dtheta1 : Outport  Port=3
  theta2 : Outport  Port=4
  theta3 : Outport  Port=5
  pos2 : Outport  Port=6
  dtheta2 : Outport  Port=7
  dtheta3 : Outport  Port=8
  E2 absolute : Outport  Port=9
  wires:
  Constant2/1 -> ec_TU_ES_30/3
  Constant5/1 -> ec_TU_ES_30/6
  Constant8/1 -> ec_TU_ES_30/9
  Digital/1(Out1) -> ec_TU_ES_30/10
  Constant10/1 -> ec_TU_ES_30/11
  Constant11/1 -> ec_TU_ES_30/12
  ec_TU_ES_30/1 -> Display/1
  ec_TU_ES_30/3 -> Display2/1
  ec_TU_ES_30/5 -> Display4/1, To Workspace10/1
  ec_TU_ES_30/6 -> Display5/1
  ec_TU_ES_30/8 -> Display7/1, To Workspace8/1
  ec_TU_ES_30/9 -> dtheta2/1, To Workspace13/1, [dtheta_e1]
  ec_TU_ES_30/10 -> Display9/1, Sum8/1, Sum9/1
  ec_TU_ES_30/11 -> Display10/1
  ec_TU_ES_30/13 -> Display12/1, To Workspace9/1
  ec_TU_ES_30/15 -> Display14/1, Sum8/2, Sum9/2
  ec_TU_ES_30/16 -> Terminator4/1
  ec_TU_ES_30/17 -> Terminator3/1
  ec_TU_ES_30/18 -> Terminator2/1
  ec_TU_ES_30/19 -> Display18/1, To Workspace/1, Scope/1
  ec_TU_ES_30/20 -> Display19/1, To Workspace2/1
  ec_TU_ES_30/21 -> Display20/1, To Workspace1/1
  ec_TU_ES_30/23 -> Display22/1, Sum5/1
  ec_TU_ES_30/24 -> Display23/1, Sum7/1
  ec_TU_ES_30/25 -> Terminator1/1
  ec_TU_ES_30/26 -> Terminator/1
  ec_TU_ES_30/27 -> Display26/1
  ec_TU_ES_30/28 -> Display27/1
  tau_s3/1 -> Sum/2
  C2deg/1 -> theta1/1, Display13/1
  Extended counter2/1(c_out) -> C2deg/1
  Cosntant12/1 -> Sum/1
  Sum/1 -> Saturation/1
  Saturation/1 -> ec_TU_ES_30/2, To Workspace3/1
  (max+min)/2/1 -> Sum3/2
  Sum3/1 -> C2deg1/1
  C2deg1/1 -> S3 absolute/1, pos1/1, Abs/1, Display11/1
  Abs/1 -> Switch/2
  Constant1/1 -> Switch/1
  Constant/1 -> Switch/3
  Switch/1 -> ec_TU_ES_30/1, Display1/1
  Sum1/1 -> Saturation2/1
  Saturation2/1 -> ec_TU_ES_30/5, Display6/1
  Sum2/1 -> Saturation1/1
  Saturation1/1 -> ec_TU_ES_30/8, Display8/1
  ec_TU_ES_30/12 -> Extended counter3/1(c_in)
  Extended counter1/1(c_out) -> C2deg2/1
  Extended counter3/1(c_out) -> C2deg3/1
  C2deg2/1 -> theta2/1
  C2deg3/1 -> theta3/1
  Constant7/1 -> Sum2/2
  tau_e1/1 -> Sum4/1
  Constant9/1 -> Sum4/2
  ec_TU_ES_30/22 -> Sum3/1
  (max+min)/1/1 -> Sum5/2
  Sum5/1 -> C2deg4/1
  Abs1/1 -> Switch1/2
  Constant21/1 -> Switch1/1
  Constant20/1 -> Switch1/3
  C2deg4/1 -> E1 absolute/1, pos2/1, Abs1/1
  Switch1/1 -> ec_TU_ES_30/4, ec_TU_ES_30/7, Display3/1
  Sum6/1 -> Sum2/3, Sum1/3
  tau_e2/1 -> Sum6/1
  Constant4/1 -> Sum6/2
  Constant3/1 -> Sum1/1
  ec_TU_ES_30/4 -> Gain/1
  Gain/1 -> dtheta1/1
  C2deg5/1 -> E2 absolute/1
  (max+min)/3/1 -> Sum7/2
  Sum7/1 -> C2deg5/1
  ec_TU_ES_30/2 -> Extended counter2/1(c_in)
  ec_TU_ES_30/7 -> Extended counter1/1(c_in)
  Sum8/1 -> -Kc4/1
  -Kc4/1 -> To Workspace5/1, [tau_e1_out], To Workspace11/1
  Sum9/1 -> -Kc1/1
  -Kc1/1 -> To Workspace6/1
  ec_TU_ES_30/14 -> dtheta3/1, To Workspace7/1
  Gain1/1 -> Sum1/2, Sum2/1, To Workspace12/1
  Sum12/1 -> Gain1/1, To Workspace4/1, [tau_e1_in]
  Sum4/1 -> Sum12/1
  [tauf_e1] -> Gain4/1
  Gain4/1 -> Sum12/2

== system IdentPlanar/Board 2/Sync ==
  qm : Inport
  qabs : Inport  Port=2
  sync : Inport  Port=3
  Memory : Memory
  Memory1 : Memory
  Sum2 : Sum
  Sum6 : Sum  Inputs=+-|
  Switch : Switch  Criteria=u2 > Threshold
  Switch1 : Switch  Criteria=u2 > Threshold
  synced : Outport
  wires:
  Switch/1 -> Sum6/2, Memory/1
  Memory/1 -> Switch/3
  qm/1 -> Switch/1, Sum6/1
  Sum6/1 -> Sum2/1
  Sum2/1 -> synced/1
  sync/1 -> Switch/2, Switch1/2
  Memory1/1 -> Switch1/3, Sum2/2
  Switch1/1 -> Memory1/1
  qabs/1 -> Switch1/1

== system IdentPlanar/Board 2/Sync1 ==
  qm : Inport
  qabs : Inport  Port=2
  sync : Inport  Port=3
  Memory : Memory
  Memory1 : Memory
  Sum2 : Sum
  Sum6 : Sum  Inputs=+-|
  Switch : Switch  Criteria=u2 > Threshold
  Switch1 : Switch  Criteria=u2 > Threshold
  synced : Outport
  wires:
  Switch/1 -> Sum6/2, Memory/1
  Memory/1 -> Switch/3
  qm/1 -> Switch/1, Sum6/1
  Sum6/1 -> Sum2/1
  Sum2/1 -> synced/1
  sync/1 -> Switch/2, Switch1/2
  Memory1/1 -> Switch1/3, Sum2/2
  Switch1/1 -> Memory1/1
  qabs/1 -> Switch1/1

== system IdentPlanar/Board 2/Sync3 ==
  qm : Inport
  qabs : Inport  Port=2
  sync : Inport  Port=3
  Memory : Memory
  Memory1 : Memory
  Sum2 : Sum
  Sum6 : Sum  Inputs=+-|
  Switch : Switch  Criteria=u2 > Threshold
  Switch1 : Switch  Criteria=u2 > Threshold
  synced : Outport
  wires:
  Switch/1 -> Sum6/2, Memory/1
  Memory/1 -> Switch/3
  qm/1 -> Switch/1, Sum6/1
  Sum6/1 -> Sum2/1
  Sum2/1 -> synced/1
  sync/1 -> Switch/2, Switch1/2
  Memory1/1 -> Switch1/3, Sum2/2
  Switch1/1 -> Memory1/1
  qabs/1 -> Switch1/1

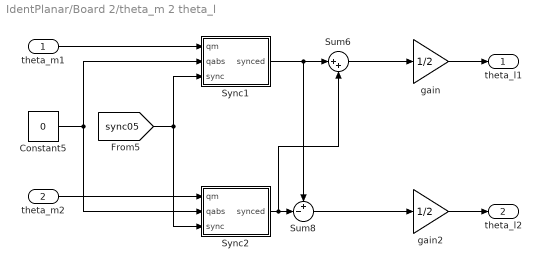
== system IdentPlanar/Board 2/theta_m 2 theta_l ==
  theta_m1 : Inport
  theta_m2 : Inport  Port=2
  Constant5 : Constant  Value=0
  Sum6 : Sum  Inputs=|++
  Sum8 : Sum  Inputs=+-|
  Sync1 : Subsystem
  Sync2 : Subsystem
  gain : Gain  Gain=1/2
  gain2 : Gain  Gain=1/2
  theta_l1 : Outport
  theta_l2 : Outport  Port=2
  wires:
  theta_m2/1 -> Sync2/1(qm)
  theta_m1/1 -> Sync1/1(qm)
  Constant5/1 -> Sync1/2(qabs), Sync2/2(qabs)
  Sync2/1(synced) -> Sum8/2, Sum6/2
  Sync1/1(synced) -> Sum6/1, Sum8/1
  Sum6/1 -> gain/1
  gain/1 -> theta_l1/1
  gain2/1 -> theta_l2/1
  [sync05] -> Sync1/3(sync), Sync2/3(sync)
  Sum8/1 -> gain2/1

== system IdentPlanar/Board 2/theta_m 2 theta_l1 ==
  theta_m1 : Inport
  theta_m2 : Inport  Port=2
  Sum6 : Sum  Inputs=|++
  Sum8 : Sum  Inputs=+-|
  gain : Gain  Gain=1/2
  gain2 : Gain  Gain=1/2
  theta_l1 : Outport
  theta_l2 : Outport  Port=2
  wires:
  Sum6/1 -> gain/1
  gain/1 -> theta_l1/1
  Sum8/1 -> gain2/1
  gain2/1 -> theta_l2/1
  theta_m1/1 -> Sum6/1, Sum8/1
  theta_m2/1 -> Sum6/2, Sum8/2

== system IdentPlanar/Board 1/Shoulder/Digital ==
  Combine_bits : Subsystem
  Constant{12..19} (8 alike) : Constant  Value=0
  Out1 : Outport
  wires:
  Constant16/1 -> Combine_bits/1(bit0)
  Constant17/1 -> Combine_bits/2(bit1)
  Constant18/1 -> Combine_bits/3(bit2)
  Constant19/1 -> Combine_bits/4(bit3)
  Constant12/1 -> Combine_bits/5(bit4)
  Constant13/1 -> Combine_bits/6(bit5)
  Constant14/1 -> Combine_bits/7(bit6)
  Constant15/1 -> Combine_bits/8(bit7)
  Combine_bits/1(Out1) -> Out1/1

== system IdentPlanar/Board 1/Shoulder/Extended counter2 ==
  c_in : Inport
  Rollover counter : Subsystem
  Sum2 : Sum  Inputs=|++
  counts per rollover : Gain  Gain=2^32
  c_out : Outport
  wires:
  counts per rollover/1 -> Sum2/1
  Rollover counter/1(Rollovers) -> counts per rollover/1
  c_in/1 -> Rollover counter/1(counts), Sum2/2
  Sum2/1 -> c_out/1

== system IdentPlanar/Board 1/Shoulder/Extended counter3 ==
  c_in : Inport
  Rollover counter : Subsystem
  Sum2 : Sum  Inputs=|++
  counts per rollover : Gain  Gain=2^32
  c_out : Outport
  wires:
  counts per rollover/1 -> Sum2/1
  Rollover counter/1(Rollovers) -> counts per rollover/1
  c_in/1 -> Rollover counter/1(counts), Sum2/2
  Sum2/1 -> c_out/1

== system IdentPlanar/Board 1/theta_m 2 theta_l/Sync1 ==
  qm : Inport
  qabs : Inport  Port=2
  sync : Inport  Port=3
  Memory : Memory
  Memory1 : Memory
  Sum2 : Sum
  Sum6 : Sum  Inputs=+-|
  Switch : Switch  Criteria=u2 > Threshold
  Switch1 : Switch  Criteria=u2 > Threshold
  synced : Outport
  wires:
  Switch/1 -> Sum6/2, Memory/1
  Memory/1 -> Switch/3
  qm/1 -> Switch/1, Sum6/1
  Sum6/1 -> Sum2/1
  Sum2/1 -> synced/1
  sync/1 -> Switch/2, Switch1/2
  Memory1/1 -> Switch1/3, Sum2/2
  Switch1/1 -> Memory1/1
  qabs/1 -> Switch1/1

== system IdentPlanar/Board 1/theta_m 2 theta_l/Sync2 ==
  qm : Inport
  qabs : Inport  Port=2
  sync : Inport  Port=3
  Memory : Memory
  Memory1 : Memory
  Sum2 : Sum
  Sum6 : Sum  Inputs=+-|
  Switch : Switch  Criteria=u2 > Threshold
  Switch1 : Switch  Criteria=u2 > Threshold
  synced : Outport
  wires:
  Switch/1 -> Sum6/2, Memory/1
  Memory/1 -> Switch/3
  qm/1 -> Switch/1, Sum6/1
  Sum6/1 -> Sum2/1
  Sum2/1 -> synced/1
  sync/1 -> Switch/2, Switch1/2
  Memory1/1 -> Switch1/3, Sum2/2
  Switch1/1 -> Memory1/1
  qabs/1 -> Switch1/1

== system IdentPlanar/Board 2/Elbow/Digital ==
  Combine_bits : Subsystem
  Constant{12..19} (8 alike) : Constant  Value=0
  Out1 : Outport
  wires:
  Constant16/1 -> Combine_bits/1(bit0)
  Constant17/1 -> Combine_bits/2(bit1)
  Constant18/1 -> Combine_bits/3(bit2)
  Constant19/1 -> Combine_bits/4(bit3)
  Constant12/1 -> Combine_bits/5(bit4)
  Constant13/1 -> Combine_bits/6(bit5)
  Constant14/1 -> Combine_bits/7(bit6)
  Constant15/1 -> Combine_bits/8(bit7)
  Combine_bits/1(Out1) -> Out1/1

== system IdentPlanar/Board 2/Elbow/Extended counter1 ==
  c_in : Inport
  Rollover counter : Subsystem
  Sum2 : Sum  Inputs=|++
  counts per rollover : Gain  Gain=2^32
  c_out : Outport
  wires:
  counts per rollover/1 -> Sum2/1
  Rollover counter/1(Rollovers) -> counts per rollover/1
  c_in/1 -> Rollover counter/1(counts), Sum2/2
  Sum2/1 -> c_out/1

== system IdentPlanar/Board 2/Elbow/Extended counter2 ==
  c_in : Inport
  Rollover counter : Subsystem
  Sum2 : Sum  Inputs=|++
  counts per rollover : Gain  Gain=2^32
  c_out : Outport
  wires:
  counts per rollover/1 -> Sum2/1
  Rollover counter/1(Rollovers) -> counts per rollover/1
  c_in/1 -> Rollover counter/1(counts), Sum2/2
  Sum2/1 -> c_out/1

== system IdentPlanar/Board 2/Elbow/Extended counter3 ==
  c_in : Inport
  Rollover counter : Subsystem
  Sum2 : Sum  Inputs=|++
  counts per rollover : Gain  Gain=2^32
  c_out : Outport
  wires:
  counts per rollover/1 -> Sum2/1
  Rollover counter/1(Rollovers) -> counts per rollover/1
  c_in/1 -> Rollover counter/1(counts), Sum2/2
  Sum2/1 -> c_out/1

== system IdentPlanar/Board 2/theta_m 2 theta_l/Sync1 ==
  qm : Inport
  qabs : Inport  Port=2
  sync : Inport  Port=3
  Memory : Memory
  Memory1 : Memory
  Sum2 : Sum
  Sum6 : Sum  Inputs=+-|
  Switch : Switch  Criteria=u2 > Threshold
  Switch1 : Switch  Criteria=u2 > Threshold
  synced : Outport
  wires:
  Switch/1 -> Sum6/2, Memory/1
  Memory/1 -> Switch/3
  qm/1 -> Switch/1, Sum6/1
  Sum6/1 -> Sum2/1
  Sum2/1 -> synced/1
  sync/1 -> Switch/2, Switch1/2
  Memory1/1 -> Switch1/3, Sum2/2
  Switch1/1 -> Memory1/1
  qabs/1 -> Switch1/1

== system IdentPlanar/Board 2/theta_m 2 theta_l/Sync2 ==
  qm : Inport
  qabs : Inport  Port=2
  sync : Inport  Port=3
  Memory : Memory
  Memory1 : Memory
  Sum2 : Sum
  Sum6 : Sum  Inputs=+-|
  Switch : Switch  Criteria=u2 > Threshold
  Switch1 : Switch  Criteria=u2 > Threshold
  synced : Outport
  wires:
  Switch/1 -> Sum6/2, Memory/1
  Memory/1 -> Switch/3
  qm/1 -> Switch/1, Sum6/1
  Sum6/1 -> Sum2/1
  Sum2/1 -> synced/1
  sync/1 -> Switch/2, Switch1/2
  Memory1/1 -> Switch1/3, Sum2/2
  Switch1/1 -> Memory1/1
  qabs/1 -> Switch1/1

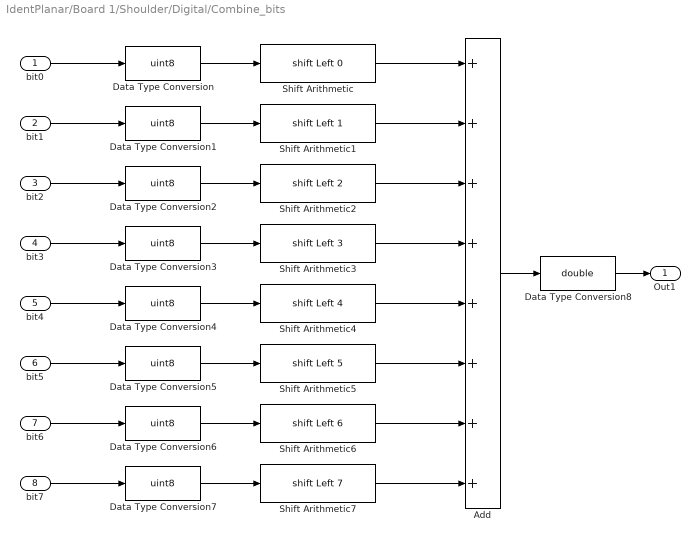
== system IdentPlanar/Board 1/Shoulder/Digital/Combine_bits ==
  bit0 : Inport
  bit1 : Inport  Port=2
  bit2 : Inport  Port=3
  bit3 : Inport  Port=4
  bit4 : Inport  Port=5
  bit5 : Inport  Port=6
  bit6 : Inport  Port=7
  bit7 : Inport  Port=8
  Add : Sum  Inputs=++++++++
  Data Type Conversion{,1..7} (8 alike) : DataTypeConversion  OutDataTypeStr=uint8
  Data Type Conversion8 : DataTypeConversion  OutDataTypeStr=double
  Shift Arithmetic : ArithShift  BitShiftDirection=Left
  Shift Arithmetic1 : ArithShift  BitShiftNumber=1  BitShiftDirection=Left
  Shift Arithmetic2 : ArithShift  BitShiftNumber=2  BitShiftDirection=Left
  Shift Arithmetic3 : ArithShift  BitShiftNumber=3  BitShiftDirection=Left
  Shift Arithmetic4 : ArithShift  BitShiftNumber=4  BitShiftDirection=Left
  Shift Arithmetic5 : ArithShift  BitShiftNumber=5  BitShiftDirection=Left
  Shift Arithmetic6 : ArithShift  BitShiftNumber=6  BitShiftDirection=Left
  Shift Arithmetic7 : ArithShift  BitShiftNumber=7  BitShiftDirection=Left
  Out1 : Outport
  wires:
  bit0/1 -> Data Type Conversion/1
  bit1/1 -> Data Type Conversion1/1
  bit2/1 -> Data Type Conversion2/1
  bit3/1 -> Data Type Conversion3/1
  bit4/1 -> Data Type Conversion4/1
  bit5/1 -> Data Type Conversion5/1
  bit6/1 -> Data Type Conversion6/1
  bit7/1 -> Data Type Conversion7/1
  Data Type Conversion/1 -> Shift Arithmetic/1
  Data Type Conversion1/1 -> Shift Arithmetic1/1
  Data Type Conversion2/1 -> Shift Arithmetic2/1
  Data Type Conversion3/1 -> Shift Arithmetic3/1
  Data Type Conversion4/1 -> Shift Arithmetic4/1
  Data Type Conversion5/1 -> Shift Arithmetic5/1
  Data Type Conversion6/1 -> Shift Arithmetic6/1
  Data Type Conversion7/1 -> Shift Arithmetic7/1
  Shift Arithmetic/1 -> Add/1
  Shift Arithmetic1/1 -> Add/2
  Shift Arithmetic2/1 -> Add/3
  Shift Arithmetic3/1 -> Add/4
  Shift Arithmetic4/1 -> Add/5
  Shift Arithmetic5/1 -> Add/6
  Shift Arithmetic6/1 -> Add/7
  Shift Arithmetic7/1 -> Add/8
  Add/1 -> Data Type Conversion8/1
  Data Type Conversion8/1 -> Out1/1

== system IdentPlanar/Board 1/Shoulder/Extended counter2/Rollover counter ==
  counts : Inport
  Abs : Abs
  Direction : Signum
  Memory : Memory  X0=2^32/2  InheritSampleTime=on
  Memory1 : Memory
  No wrap : Constant  Value=0
  Sum : Sum  Inputs=+-
  Sum1 : Sum
  Switch : Switch  Threshold=(2^32)/2+50
  Rollovers : Outport
  wires:
  Memory1/1 -> Sum1/1
  Sum1/1 -> Memory1/1, Rollovers/1
  Switch/1 -> Sum1/2
  Direction/1 -> Switch/1
  No wrap/1 -> Switch/3
  Abs/1 -> Switch/2
  Sum/1 -> Abs/1, Direction/1
  Memory/1 -> Sum/1
  counts/1 -> Sum/2, Memory/1

== system IdentPlanar/Board 1/Shoulder/Extended counter3/Rollover counter ==
  counts : Inport
  Abs : Abs
  Direction : Signum
  Memory : Memory  X0=2^32/2  InheritSampleTime=on
  Memory1 : Memory
  No wrap : Constant  Value=0
  Sum : Sum  Inputs=+-
  Sum1 : Sum
  Switch : Switch  Threshold=(2^32)/2+50
  Rollovers : Outport
  wires:
  Memory1/1 -> Sum1/1
  Sum1/1 -> Memory1/1, Rollovers/1
  Switch/1 -> Sum1/2
  Direction/1 -> Switch/1
  No wrap/1 -> Switch/3
  Abs/1 -> Switch/2
  Sum/1 -> Abs/1, Direction/1
  Memory/1 -> Sum/1
  counts/1 -> Sum/2, Memory/1

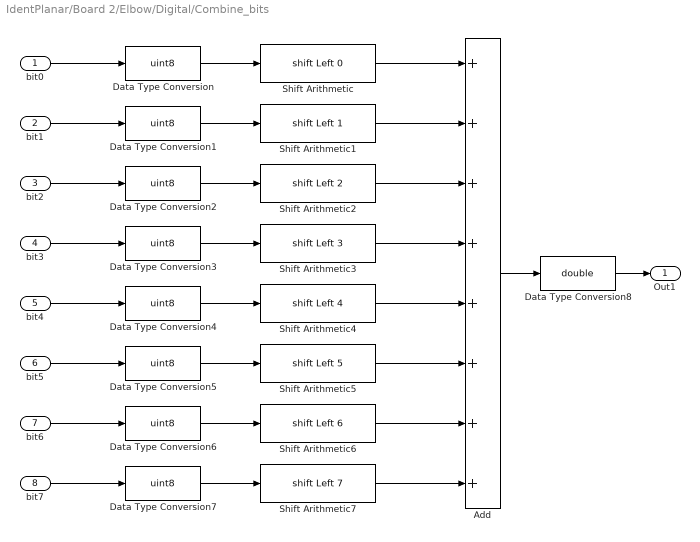
== system IdentPlanar/Board 2/Elbow/Digital/Combine_bits ==
  bit0 : Inport
  bit1 : Inport  Port=2
  bit2 : Inport  Port=3
  bit3 : Inport  Port=4
  bit4 : Inport  Port=5
  bit5 : Inport  Port=6
  bit6 : Inport  Port=7
  bit7 : Inport  Port=8
  Add : Sum  Inputs=++++++++
  Data Type Conversion{,1..7} (8 alike) : DataTypeConversion  OutDataTypeStr=uint8
  Data Type Conversion8 : DataTypeConversion  OutDataTypeStr=double
  Shift Arithmetic : ArithShift  BitShiftDirection=Left
  Shift Arithmetic1 : ArithShift  BitShiftNumber=1  BitShiftDirection=Left
  Shift Arithmetic2 : ArithShift  BitShiftNumber=2  BitShiftDirection=Left
  Shift Arithmetic3 : ArithShift  BitShiftNumber=3  BitShiftDirection=Left
  Shift Arithmetic4 : ArithShift  BitShiftNumber=4  BitShiftDirection=Left
  Shift Arithmetic5 : ArithShift  BitShiftNumber=5  BitShiftDirection=Left
  Shift Arithmetic6 : ArithShift  BitShiftNumber=6  BitShiftDirection=Left
  Shift Arithmetic7 : ArithShift  BitShiftNumber=7  BitShiftDirection=Left
  Out1 : Outport
  wires:
  bit0/1 -> Data Type Conversion/1
  bit1/1 -> Data Type Conversion1/1
  bit2/1 -> Data Type Conversion2/1
  bit3/1 -> Data Type Conversion3/1
  bit4/1 -> Data Type Conversion4/1
  bit5/1 -> Data Type Conversion5/1
  bit6/1 -> Data Type Conversion6/1
  bit7/1 -> Data Type Conversion7/1
  Data Type Conversion/1 -> Shift Arithmetic/1
  Data Type Conversion1/1 -> Shift Arithmetic1/1
  Data Type Conversion2/1 -> Shift Arithmetic2/1
  Data Type Conversion3/1 -> Shift Arithmetic3/1
  Data Type Conversion4/1 -> Shift Arithmetic4/1
  Data Type Conversion5/1 -> Shift Arithmetic5/1
  Data Type Conversion6/1 -> Shift Arithmetic6/1
  Data Type Conversion7/1 -> Shift Arithmetic7/1
  Shift Arithmetic/1 -> Add/1
  Shift Arithmetic1/1 -> Add/2
  Shift Arithmetic2/1 -> Add/3
  Shift Arithmetic3/1 -> Add/4
  Shift Arithmetic4/1 -> Add/5
  Shift Arithmetic5/1 -> Add/6
  Shift Arithmetic6/1 -> Add/7
  Shift Arithmetic7/1 -> Add/8
  Add/1 -> Data Type Conversion8/1
  Data Type Conversion8/1 -> Out1/1

== system IdentPlanar/Board 2/Elbow/Extended counter1/Rollover counter ==
  counts : Inport
  Abs : Abs
  Direction : Signum
  Memory : Memory  X0=2^32/2  InheritSampleTime=on
  Memory1 : Memory
  No wrap : Constant  Value=0
  Sum : Sum  Inputs=+-
  Sum1 : Sum
  Switch : Switch  Threshold=(2^32)/2+50
  Rollovers : Outport
  wires:
  Memory1/1 -> Sum1/1
  Sum1/1 -> Memory1/1, Rollovers/1
  Switch/1 -> Sum1/2
  Direction/1 -> Switch/1
  No wrap/1 -> Switch/3
  Abs/1 -> Switch/2
  Sum/1 -> Abs/1, Direction/1
  Memory/1 -> Sum/1
  counts/1 -> Sum/2, Memory/1

== system IdentPlanar/Board 2/Elbow/Extended counter2/Rollover counter ==
  counts : Inport
  Abs : Abs
  Direction : Signum
  Memory : Memory  X0=2^32/2  InheritSampleTime=on
  Memory1 : Memory
  No wrap : Constant  Value=0
  Sum : Sum  Inputs=+-
  Sum1 : Sum
  Switch : Switch  Threshold=(2^32)/2+50
  Rollovers : Outport
  wires:
  Memory1/1 -> Sum1/1
  Sum1/1 -> Memory1/1, Rollovers/1
  Switch/1 -> Sum1/2
  Direction/1 -> Switch/1
  No wrap/1 -> Switch/3
  Abs/1 -> Switch/2
  Sum/1 -> Abs/1, Direction/1
  Memory/1 -> Sum/1
  counts/1 -> Sum/2, Memory/1

== system IdentPlanar/Board 2/Elbow/Extended counter3/Rollover counter ==
  counts : Inport
  Abs : Abs
  Direction : Signum
  Memory : Memory  X0=2^32/2  InheritSampleTime=on
  Memory1 : Memory
  No wrap : Constant  Value=0
  Sum : Sum  Inputs=+-
  Sum1 : Sum
  Switch : Switch  Threshold=(2^32)/2+50
  Rollovers : Outport
  wires:
  Memory1/1 -> Sum1/1
  Sum1/1 -> Memory1/1, Rollovers/1
  Switch/1 -> Sum1/2
  Direction/1 -> Switch/1
  No wrap/1 -> Switch/3
  Abs/1 -> Switch/2
  Sum/1 -> Abs/1, Direction/1
  Memory/1 -> Sum/1
  counts/1 -> Sum/2, Memory/1

== matlab function Gravity Compensation/MATLAB Function ==
  data: tau_g1 output double; tau_g2 output double; tau_g3 output double; consts input double; s1 input double; tau_g4 output double; s2 input double; s3 input double; e1 input double; e2 input double
function [tau_g1, tau_g2, tau_g3, tau_g4]  = gravcomp(consts,s1,s2,s3,e1,e2)
%% Calculates gravity compensation torques for each DOF
% Consts:
% 1: deg_rad
% 2: Lu
% 3: mu
% 4: Ll
% 5: ml

% 6: c1x
% 7: c1y
% 8: c1z
% 9: c2x
% 10: c2y
% 11: c2z
% 12: c3x
% 13: c3y
% 14: c3z
% 15: c4x
% 16: c4y
% 17: c4z
% 18: c5x
% 19: c5y
% 20: c5z

% 21: Nm2mA_s1
% 22: Nm2mA_s2
% 23: Nm2mA_s3
% 24: Nm2mA_e1

Lu = consts(2);
mu = consts(3);
Ll = consts(4);
ml = consts(5);
mw = 0;
Lw = 0;

%% Convert DOF from degrees to radians.
th1 = s1*consts(1);
th2 = s2*consts(1)-pi/2;
th3 = s3*consts(1);
th4 = e1*consts(1);
th5 = e2*consts(1);
th6 = 0;
th7 = 0;

%% Calculate trigonometric funcions once for faster calculation
c1 = cos(th1); s1 = sin(th1);
c2 = cos(th2); s2 = sin(th2);
c3 = cos(th3); s3 = sin(th3);
c4 = cos(th4); s4 = sin(th4);
c5 = cos(th5); s5 = sin(th5);
c6 = cos(th6); s6 = sin(th6);
c7 = cos(th7); s7 = sin(th7);

%% COGs
c1x = consts(6); c1y = consts(7); c1z = consts(8);
c2x = consts(9); c2y = consts(10); c2z = consts(11);
c3x = consts(12); c3y = consts(13); c3z = consts(14);
c4x = consts(15); c4y = consts(16); c4z = consts(17);
c5x = consts(18); c5y = consts(19); c5z = consts(20);
c6x = 0; c6y = 0; c6z = 0;
c7x = 0; c7y = 0; c7z = 0;

%% Calculate torques resulting from gravity (run ownmodel.m to find formulas)
tau_g1Nm = (981*ml*(c4y*(c1*c3 - c2*s1*s3) + c4x*(c4*(c1*s3 + c2*c3*s1) - s1*s2*s4) + c4z*(s4*(c1*s3 + c2*c3*s1) + c4*s1*s2) + Lu*s1*s2))/100 - (981*mw*(c7y*(c6*(s4*(c1*s3 + c2*c3*s1) + c4*s1*s2) + s6*(c5*(c4*(c1*s3 + c2*c3*s1) - s1*s2*s4) + s5*(c1*c3 - c2*s1*s3))) + c7x*(c7*(s6*(s4*(c1*s3 + c2*c3*s1) + c4*s1*s2) - c6*(c5*(c4*(c1*s3 + c2*c3*s1) - s1*s2*s4) + s5*(c1*c3 - c2*s1*s3))) + s7*(s5*(c4*(c1*s3 + c2*c3*s1) - s1*s2*s4) - c5*(c1*c3 - c2*s1*s3))) + c7z*(c7*(s5*(c4*(c1*s3 + c2*c3*s1) - s1*s2*s4) - c5*(c1*c3 - c2*s1*s3)) - s7*(s6*(s4*(c1*s3 + c2*c3*s1) + c4*s1*s2) - c6*(c5*(c4*(c1*s3 + c2*c3*s1) - s1*s2*s4) + s5*(c1*c3 - c2*s1*s3)))) - Ll*(s4*(c1*s3 + c2*c3*s1) + c4*s1*s2) + Lw*s7*(s5*(c4*(c1*s3 + c2*c3*s1) - s1*s2*s4) - c5*(c1*c3 - c2*s1*s3)) - Lu*s1*s2 + Lw*c7*(s6*(s4*(c1*s3 + c2*c3*s1) + c4*s1*s2) - c6*(c5*(c4*(c1*s3 + c2*c3*s1) - s1*s2*s4) + s5*(c1*c3 - c2*s1*s3)))))/100 + (981*mu*(c2y*c1 + c2x*c2*s1 + c2z*s1*s2))/100;

tau_g2Nm = -(981*mu*(c2z*c1*c2 - c2x*c1*s2))/100 - (981*mw*(Ll*(c1*c2*c4 - c1*c3*s2*s4) - c7y*(c6*(c1*c2*c4 - c1*c3*s2*s4) - s6*(c5*(c1*c2*s4 + c1*c3*c4*s2) - c1*s2*s3*s5)) - c7x*(c7*(s6*(c1*c2*c4 - c1*c3*s2*s4) + c6*(c5*(c1*c2*s4 + c1*c3*c4*s2) - c1*s2*s3*s5)) - s7*(s5*(c1*c2*s4 + c1*c3*c4*s2) + c1*c5*s2*s3)) + c7z*(c7*(s5*(c1*c2*s4 + c1*c3*c4*s2) + c1*c5*s2*s3) + s7*(s6*(c1*c2*c4 - c1*c3*s2*s4) + c6*(c5*(c1*c2*s4 + c1*c3*c4*s2) - c1*s2*s3*s5))) - Lw*c7*(s6*(c1*c2*c4 - c1*c3*s2*s4) + c6*(c5*(c1*c2*s4 + c1*c3*c4*s2) - c1*s2*s3*s5)) + Lw*s7*(s5*(c1*c2*s4 + c1*c3*c4*s2) + c1*c5*s2*s3) + Lu*c1*c2))/100 - (981*ml*(c4z*(c1*c2*c4 - c1*c3*s2*s4) - c4x*(c1*c2*s4 + c1*c3*c4*s2) + Lu*c1*c2 + c4y*c1*s2*s3))/100;
tau_g3Nm = (981*ml*(c4x*c4*(c3*s1 + c1*c2*s3) - c4y*(s1*s3 - c1*c2*c3) + c4z*s4*(c3*s1 + c1*c2*s3)))/100 - (981*mw*(c7x*(c7*(c6*(s5*(s1*s3 - c1*c2*c3) - c4*c5*(c3*s1 + c1*c2*s3)) + s4*s6*(c3*s1 + c1*c2*s3)) + s7*(c5*(s1*s3 - c1*c2*c3) + c4*s5*(c3*s1 + c1*c2*s3))) - c7z*(s7*(c6*(s5*(s1*s3 - c1*c2*c3) - c4*c5*(c3*s1 + c1*c2*s3)) + s4*s6*(c3*s1 + c1*c2*s3)) - c7*(c5*(s1*s3 - c1*c2*c3) + c4*s5*(c3*s1 + c1*c2*s3))) - c7y*(s6*(s5*(s1*s3 - c1*c2*c3) - c4*c5*(c3*s1 + c1*c2*s3)) - c6*s4*(c3*s1 + c1*c2*s3)) - Ll*s4*(c3*s1 + c1*c2*s3) + Lw*s7*(c5*(s1*s3 - c1*c2*c3) + c4*s5*(c3*s1 + c1*c2*s3)) + Lw*c7*(c6*(s5*(s1*s3 - c1*c2*c3) - c4*c5*(c3*s1 + c1*c2*s3)) + s4*s6*(c3*s1 + c1*c2*s3))))/100;
tau_g4Nm = - (981*mw*(c7x*(c7*(s6*(c4*(s1*s3 - c1*c2*c3) + c1*s2*s4) + c5*c6*(s4*(s1*s3 - c1*c2*c3) - c1*c4*s2)) - s5*s7*(s4*(s1*s3 - c1*c2*c3) - c1*c4*s2)) - c7z*(s7*(s6*(c4*(s1*s3 - c1*c2*c3) + c1*s2*s4) + c5*c6*(s4*(s1*s3 - c1*c2*c3) - c1*c4*s2)) + c7*s5*(s4*(s1*s3 - c1*c2*c3) - c1*c4*s2)) + c7y*(c6*(c4*(s1*s3 - c1*c2*c3) + c1*s2*s4) - c5*s6*(s4*(s1*s3 - c1*c2*c3) - c1*c4*s2)) - Ll*(c4*(s1*s3 - c1*c2*c3) + c1*s2*s4) + Lw*c7*(s6*(c4*(s1*s3 - c1*c2*c3) + c1*s2*s4) + c5*c6*(s4*(s1*s3 - c1*c2*c3) - c1*c4*s2)) - Lw*s5*s7*(s4*(s1*s3 - c1*c2*c3) - c1*c4*s2)))/100 - (981*ml*(c4x*(s4*(s1*s3 - c1*c2*c3) - c1*c4*s2) - c4z*(c4*(s1*s3 - c1*c2*c3) + c1*s2*s4)))/100;

%% Convert from Nm to mA 
tau_g1 = consts(21)*tau_g1Nm;
tau_g2 = consts(22)*tau_g2Nm;
tau_g3 = consts(23)*tau_g3Nm;
tau_g4 = consts(24)*tau_g4Nm;
end
